simulink model "WashoutFilter"  (R2019b)
settings: Solver=VariableStepAuto  StartTime=0.0  StopTime=42  RelTol=1e-3
values from neighbouring files (symbols this model uses):
  Cf = 160000    [Advance_Filters_Task2.m]    (also in Basic_Filters_Task1.m; Init_for_washout_filter.m; UKF_Task2b.m = 140000; UKF_Task2c.m)
  Cr = 225000    [Advance_Filters_Task2.m]    (also in Basic_Filters_Task1.m; Init_for_washout_filter.m; UKF_Task2b.m; UKF_Task2c.m)
  lf = 1.65    [Advance_Filters_Task2.m]    (also in Basic_Filters_Task1.m; Init_for_washout_filter.m; UKF_Task2b.m; UKF_Task2c.m)
  lr = L-lf    (= 1.291)    [Advance_Filters_Task2.m]    (also in Basic_Filters_Task1.m; Init_for_washout_filter.m; UKF_Task2b.m; UKF_Task2c.m)
  mass = 2010.5    [Advance_Filters_Task2.m]    (also in Basic_Filters_Task1.m; Init_for_washout_filter.m; UKF_Task2b.m; UKF_Task2c.m)
  rx = 0.29    [Advance_Filters_Task2.m]    (also in Basic_Filters_Task1.m; Init_for_washout_filter.m; UKF_Task2b.m; UKF_Task2c.m)
  ry = 0    [Advance_Filters_Task2.m]    (also in Basic_Filters_Task1.m; Init_for_washout_filter.m; UKF_Task2b.m; UKF_Task2c.m)
libraries: simulink x1
settings Model: Creator=Hp  LastModifiedBy=Hp

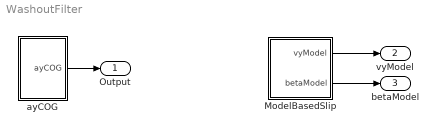
== system WashoutFilter ==
  ModelBasedSlip : Subsystem
  ayCOG : Subsystem
  Output : Outport
  vyModel : Outport  Port=2
  betaModel : Outport  Port=3
  wires:
  ayCOG/1(ayCOG) -> Output/1
  ModelBasedSlip/1(vyModel) -> vyModel/1
  ModelBasedSlip/2(betaModel) -> betaModel/1

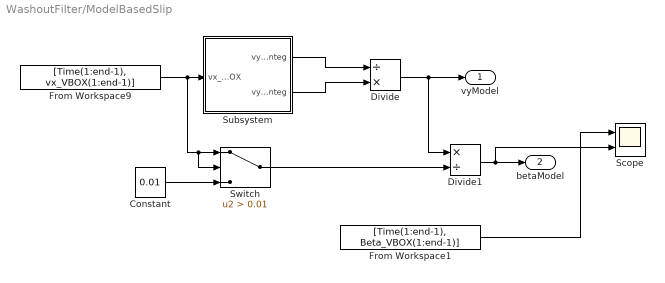
== system WashoutFilter/ModelBasedSlip ==
  Constant : Constant  Value=0.01
  Divide : Product  Inputs=/*
  Divide1 : Product  Inputs=*/
  From Workspace1 : FromWorkspace  VariableName=[Time(1:end-1), Beta_VBOX(1:end-1)]
  From Workspace9 : FromWorkspace  VariableName=[Time(1:end-1), vx_VBOX(1:end-1)]
  Scope : Scope  NumInputPorts=2
  Subsystem : Subsystem
  Switch : Switch  Criteria=u2 > Threshold  Threshold=0.01
  vyModel : Outport
  betaModel : Outport  Port=2
  wires:
  Switch/1 -> Divide1/2
  Divide1/1 -> betaModel/1, Scope/2
  From Workspace9/1 -> Switch/2, Switch/1, Subsystem/1("vx_VBOX ")
  Subsystem/1(vyDenomInteg) -> Divide/1
  Divide/1 -> vyModel/1, Divide1/1
  From Workspace1/1 -> Scope/1
  Constant/1 -> Switch/3
  Subsystem/2(vyNumInteg) -> Divide/2

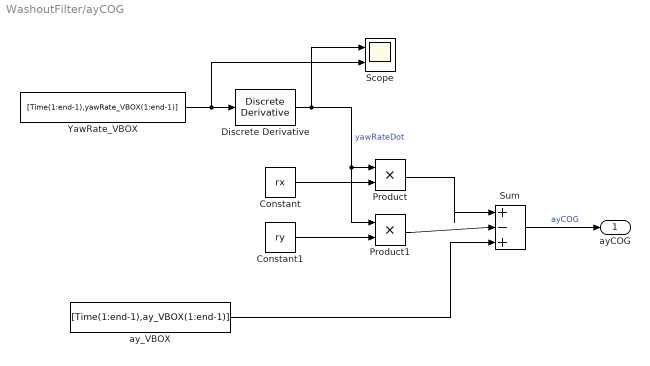
== system WashoutFilter/ayCOG ==
  Constant : Constant  Value=rx
  Constant1 : Constant  Value=ry
  Discrete Derivative : simulink/Discrete/Discrete Derivative  gainval=1.0  ICPrevScaledInput=0.0  OutMin=[]  OutMax=[]  OutDataType=fixdt(1, 16)  OutScaling=2^-10  DoSatur=off
  Product : Product
  Product1 : Product
  Scope : Scope  NumInputPorts=2
  Sum : Sum  Inputs=|+-+
  YawRate_VBOX : FromWorkspace  VariableName=[Time(1:end-1),yawRate_VBOX(1:end-1)]
  ay_VBOX : FromWorkspace  VariableName=[Time(1:end-1),ay_VBOX(1:end-1)]
  ayCOG : Outport
  wires:
  Sum/1 -> ayCOG/1  "ayCOG"
  Constant/1 -> Product/2
  YawRate_VBOX/1 -> Scope/2, Discrete Derivative/1
  Product1/1 -> Sum/2
  Product/1 -> Sum/1
  Discrete Derivative/1 -> Scope/1, Product1/1, Product/1  "yawRateDot"
  ay_VBOX/1 -> Sum/3
  Constant1/1 -> Product1/2

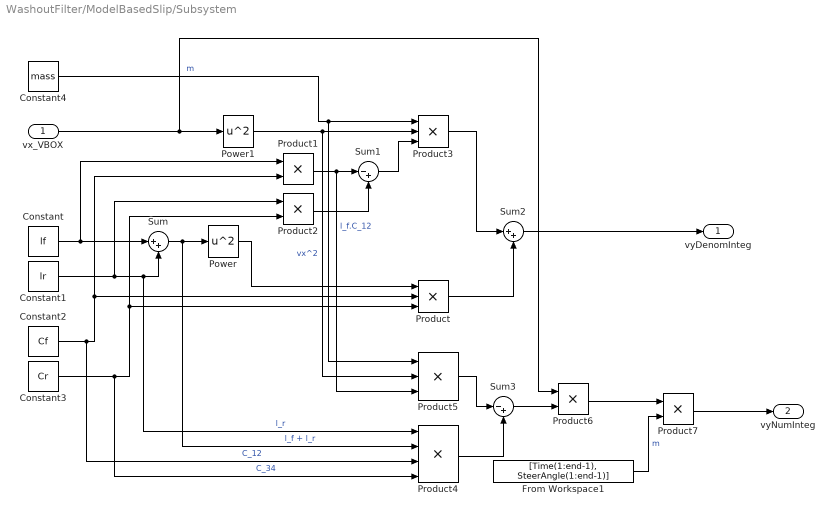
== system WashoutFilter/ModelBasedSlip/Subsystem ==
  "vx_VBOX " : Inport
  Constant : Constant  Value=lf
  Constant1 : Constant  Value=lr
  Constant2 : Constant  Value=Cf
  Constant3 : Constant  Value=Cr
  Constant4 : Constant  Value=mass
  From Workspace1 : FromWorkspace  VariableName=[Time(1:end-1), SteerAngle(1:end-1)]
  Power : Math  Operator=square  SignedPower=off  SaturateOnIntegerOverflow=on
  Power1 : Math  Operator=square  SignedPower=off  SaturateOnIntegerOverflow=on
  Product : Product  Inputs=3
  Product{1..2,6..7} (4 alike) : Product
  Product3 : Product  Inputs=3
  Product4 : Product  Inputs=4
  Product5 : Product  Inputs=3
  Sum : Sum  Inputs=|++
  Sum1 : Sum  Inputs=|-+
  Sum2 : Sum  Inputs=|++
  Sum3 : Sum  Inputs=|-+
  vyDenomInteg : Outport
  vyNumInteg : Outport  Port=2
  wires:
  Constant4/1 -> Product5/1, Product3/1  "m"
  Sum/1 -> Product4/2, Power/1  "l_f + l_r"
  Constant1/1 -> Product2/1, Product4/1, Sum/2  "l_r"
  Constant2/1 -> Product4/3, Product1/2, Product/2  "C_12"
  Constant3/1 -> Product4/4, Product2/2, Product/3  "C_34"
  Product1/1 -> Product5/3, Sum1/1  "l_f.C_12"
  Constant/1 -> Sum/1, Product1/1
  Sum2/1 -> vyDenomInteg/1
  Power1/1 -> Product5/2, Product3/2  "vx^2"
  Sum3/1 -> Product6/2
  From Workspace1/1 -> Product7/2  "m"
  Product6/1 -> Product7/1
  Sum1/1 -> Product3/3
  Product3/1 -> Sum2/1
  "vx_VBOX "/1 -> Product6/1, Power1/1
  Product7/1 -> vyNumInteg/1
  Product4/1 -> Sum3/2
  Product/1 -> Sum2/2
  Product2/1 -> Sum1/2
  Power/1 -> Product/1
  Product5/1 -> Sum3/1
